simulink model "Power_split_controller"  (R2021b)
settings: Solver=VariableStepAuto  StartTime=0.0  StopTime=274  RelTol=1
undefined symbols (not defined in the file): ISOC_sy, Pd_SY, Pl_sy, Pu_sy, QC_sy, R0_sy, SOC_H, SOC_L, V0_sy
libraries: simulink x1
settings Model: Creator=bldha  LastModifiedBy=bldha
settings SolverCC: ZeroCrossAlgorithm=Adaptive
settings DebuggingCC: IgnoredZcDiagnostic=none

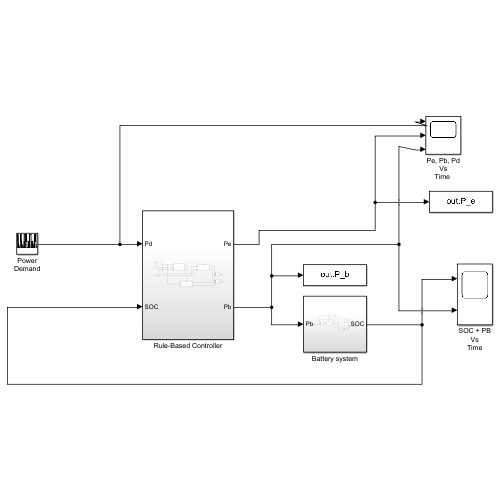
[thumbnail: Simulink's stored preview of the top-level diagram]
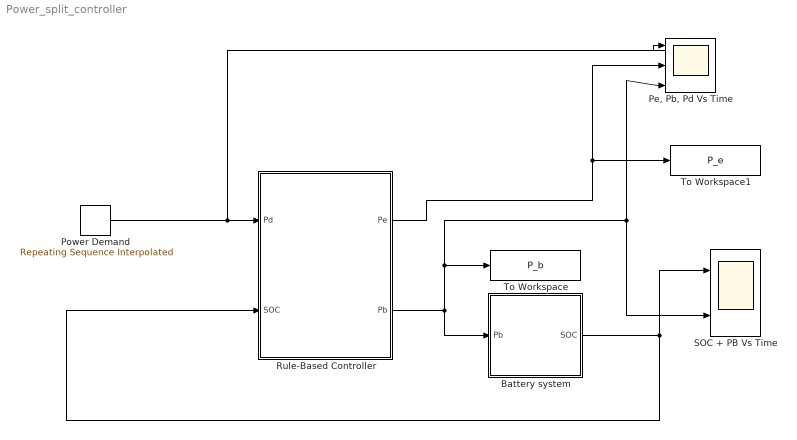
== system Power_split_controller ==
  Battery system : Subsystem
  "Pe, Pb, Pd Vs Time " : Scope  NumInputPorts=3
  Power Demand : simulink/Sources/Repeating Sequence Interpolated  OutValues=[Pd_SY.pow]  TimeValues=[Pd_SY.time]  LookUpMeth=Interpolation-Use End Values  tsamp=0.1  OutMin=[]  OutMax=[]  OutDataTypeStr=double  OutputDataTypeScalingMode=double  OutDataType=fixdt(0,8)  OutScaling=2^-10
  Rule-Based Controller : Subsystem
  SOC + PB Vs Time : Scope  NumInputPorts=2
  To Workspace : ToWorkspace  VariableName=P_b  SampleTime=-1
  To Workspace1 : ToWorkspace  VariableName=P_e  SampleTime=-1
  wires:
  Battery system/1(SOC) -> SOC + PB Vs Time/1, Rule-Based Controller/2(SOC)
  Rule-Based Controller/1(Pe) -> "Pe, Pb, Pd Vs Time "/2, To Workspace1/1
  Power Demand/1 -> Rule-Based Controller/1(Pd), "Pe, Pb, Pd Vs Time "/1
  Rule-Based Controller/2(Pb) -> To Workspace/1, "Pe, Pb, Pd Vs Time "/3, SOC + PB Vs Time/2, Battery system/1(Pb)

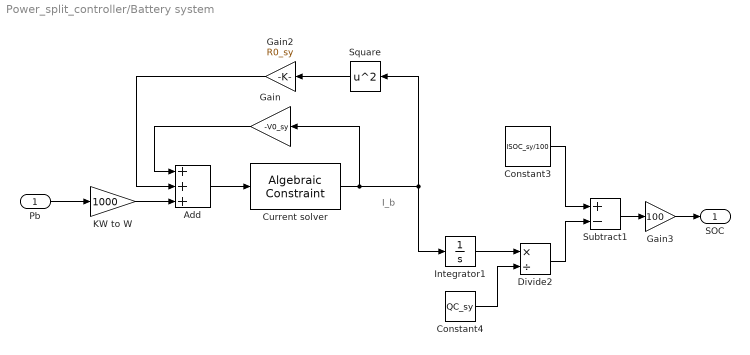
== system Power_split_controller/Battery system ==
  note: I_b
  Pb : Inport
  Add : Sum  Inputs=+++
  Constant3 : Constant  Value=ISOC_sy/100
  Constant4 : Constant  Value=QC_sy
  Current solver : AlgebraicConstraint  InitialGuess=-999999999999
  Divide2 : Product  Inputs=*/
  Gain : Gain  Gain=-V0_sy
  Gain2 : Gain  Gain=R0_sy
  Gain3 : Gain  Gain=100
  Integrator1 : Integrator
  KW to W : Gain  Gain=1000
  Square : Math  Operator=square  SaturateOnIntegerOverflow=on
  Subtract1 : Sum  Inputs=+-
  SOC : Outport
  wires:
  KW to W/1 -> Add/3
  Gain/1 -> Add/1
  Add/1 -> Current solver/1
  Square/1 -> Gain2/1
  Gain2/1 -> Add/2
  Pb/1 -> KW to W/1
  Divide2/1 -> Subtract1/2
  Constant3/1 -> Subtract1/1
  Subtract1/1 -> Gain3/1
  Gain3/1 -> SOC/1
  Current solver/1 -> Gain/1, Square/1, Integrator1/1
  Integrator1/1 -> Divide2/1
  Constant4/1 -> Divide2/2

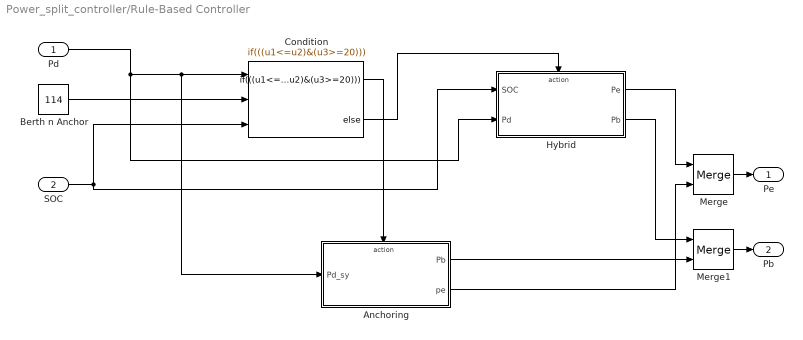
== system Power_split_controller/Rule-Based Controller ==
  Pd : Inport
  SOC : Inport  Port=2
  Anchoring : Subsystem  TreatAsAtomicUnit=on
  Berth n Anchor : Constant  Value=114
  Condition : If  NumInputs=3  IfExpression=((u1<=u2)&(u3>=20))
  Hybrid : Subsystem  TreatAsAtomicUnit=on
  Merge : Merge
  Merge1 : Merge
  Pe : Outport
  Pb : Outport  Port=2
  wires:
  Merge/1 -> Pe/1
  Pd/1 -> Hybrid/2(Pd), Anchoring/1(Pd_sy), Condition/1
  Berth n Anchor/1 -> Condition/2
  Anchoring/1(Pb) -> Merge1/2
  Hybrid/2(Pb) -> Merge1/1
  Merge1/1 -> Pb/1
  Hybrid/1(Pe) -> Merge/1
  Anchoring/2(pe) -> Merge/2
  SOC/1 -> Hybrid/1(SOC), Condition/3
  Condition/1 -> Anchoring/Action
  Condition/2 -> Hybrid/Action

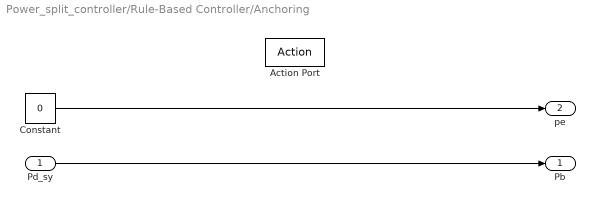
== system Power_split_controller/Rule-Based Controller/Anchoring ==
  Pd_sy : Inport
  Action Port : ActionPort  ActionPortLabel=if(((u1<=u2)&(u3>=20)))
  Constant : Constant  Value=0
  Pb : Outport
  pe : Outport  Port=2
  wires:
  Pd_sy/1 -> Pb/1
  Constant/1 -> pe/1

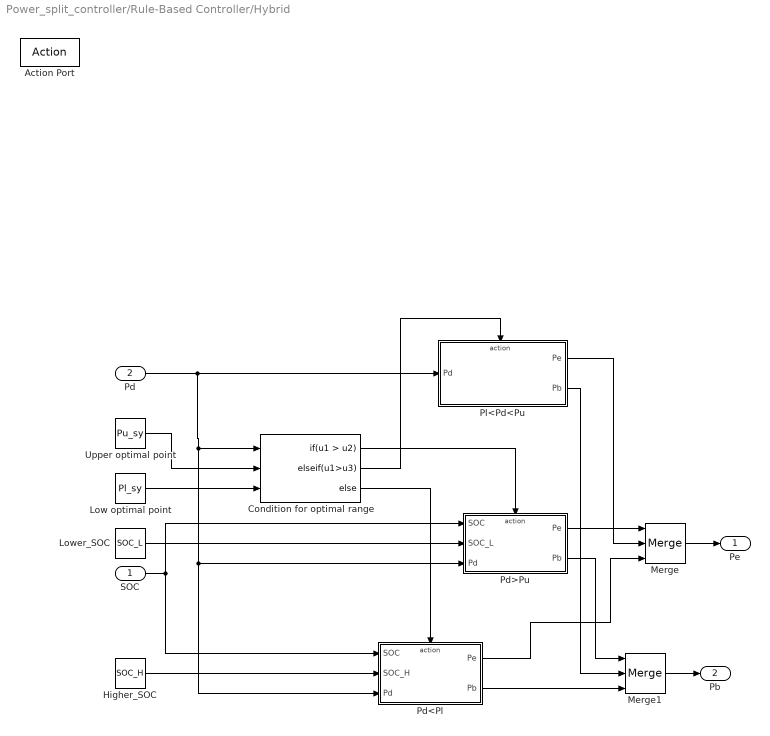
== system Power_split_controller/Rule-Based Controller/Hybrid ==
  SOC : Inport
  Pd : Inport  Port=2
  Action Port : ActionPort  ActionPortLabel=else
  "   Low optimal point" : Constant  Value=Pl_sy
  "  Upper optimal point " : Constant  Value=Pu_sy
  Condition for optimal range : If  NumInputs=3  IfExpression=u1 > u2  ElseIfExpressions=u1>u3
  Higher_SOC : Constant  Value=SOC_H
  Lower_SOC : Constant  Value=SOC_L
  Merge : Merge  Inputs=3
  Merge1 : Merge  Inputs=3
  Pd<Pl : Subsystem  TreatAsAtomicUnit=on
  Pd>Pu : Subsystem  TreatAsAtomicUnit=on
  Pl<Pd<Pu : Subsystem  TreatAsAtomicUnit=on
  Pe : Outport
  Pb : Outport  Port=2
  wires:
  Higher_SOC/1 -> Pd<Pl/2(SOC_H)
  Pl<Pd<Pu/2(Pb) -> Merge1/2
  Merge/1 -> Pe/1
  Pl<Pd<Pu/1(Pe) -> Merge/2
  Pd>Pu/2(Pb) -> Merge1/1
  Pd<Pl/1(Pe) -> Merge/3
  Lower_SOC/1 -> Pd>Pu/2(SOC_L)
  Pd/1 -> Pl<Pd<Pu/1(Pd), Pd<Pl/3(Pd), Pd>Pu/3(Pd), Condition for optimal range/1
  Condition for optimal range/2 -> Pl<Pd<Pu/Action
  Pd<Pl/2(Pb) -> Merge1/3
  "  Upper optimal point "/1 -> Condition for optimal range/2
  Condition for optimal range/3 -> Pd<Pl/Action
  Condition for optimal range/1 -> Pd>Pu/Action
  "   Low optimal point"/1 -> Condition for optimal range/3
  Pd>Pu/1(Pe) -> Merge/1
  Merge1/1 -> Pb/1
  SOC/1 -> Pd>Pu/1(SOC), Pd<Pl/1(SOC)

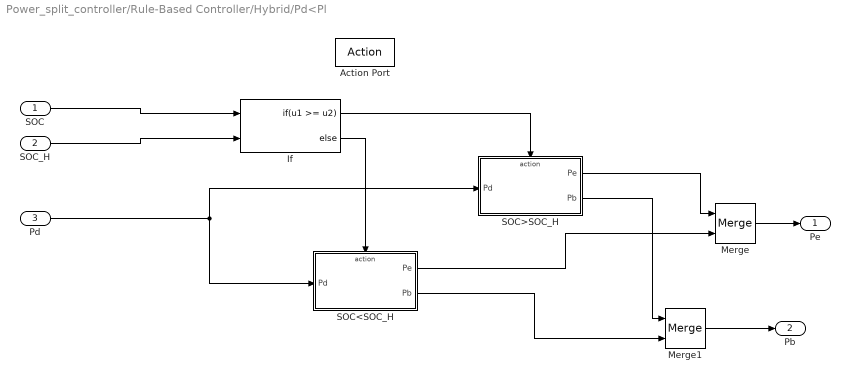
== system Power_split_controller/Rule-Based Controller/Hybrid/Pd<Pl ==
  SOC : Inport
  SOC_H : Inport  Port=2
  Pd : Inport  Port=3
  Action Port : ActionPort  ActionPortLabel=else
  If : If  NumInputs=2  IfExpression=u1 >= u2
  Merge : Merge
  Merge1 : Merge
  SOC<SOC_H : Subsystem  TreatAsAtomicUnit=on
  SOC>SOC_H : Subsystem  TreatAsAtomicUnit=on
  Pe : Outport
  Pb : Outport  Port=2
  wires:
  SOC/1 -> If/1
  SOC_H/1 -> If/2
  SOC>SOC_H/1(Pe) -> Merge/1
  SOC<SOC_H/1(Pe) -> Merge/2
  Merge/1 -> Pe/1
  SOC>SOC_H/2(Pb) -> Merge1/1
  SOC<SOC_H/2(Pb) -> Merge1/2
  Merge1/1 -> Pb/1
  Pd/1 -> SOC<SOC_H/1(Pd), SOC>SOC_H/1(Pd)
  If/2 -> SOC<SOC_H/Action
  If/1 -> SOC>SOC_H/Action

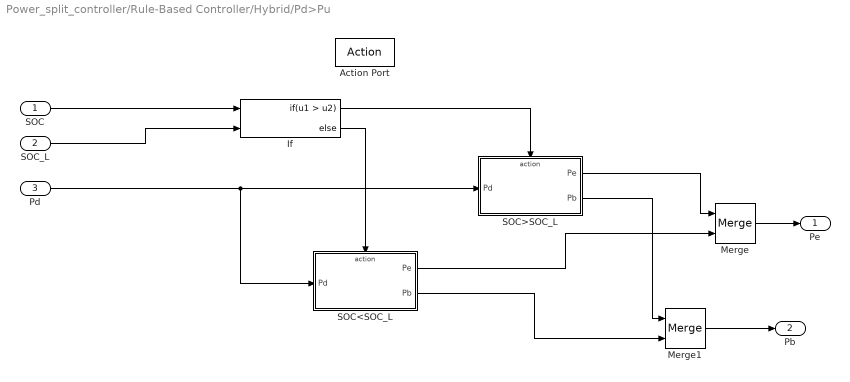
== system Power_split_controller/Rule-Based Controller/Hybrid/Pd>Pu ==
  SOC : Inport
  SOC_L : Inport  Port=2
  Pd : Inport  Port=3
  Action Port : ActionPort  ActionPortLabel=if(u1 > u2)
  If : If  NumInputs=2  IfExpression=u1 > u2
  Merge : Merge
  Merge1 : Merge
  SOC<SOC_L : Subsystem  TreatAsAtomicUnit=on
  SOC>SOC_L : Subsystem  TreatAsAtomicUnit=on
  Pe : Outport
  Pb : Outport  Port=2
  wires:
  SOC/1 -> If/1
  SOC_L/1 -> If/2
  If/1 -> SOC>SOC_L/Action
  If/2 -> SOC<SOC_L/Action
  SOC>SOC_L/1(Pe) -> Merge/1
  SOC<SOC_L/1(Pe) -> Merge/2
  Merge/1 -> Pe/1
  SOC>SOC_L/2(Pb) -> Merge1/1
  SOC<SOC_L/2(Pb) -> Merge1/2
  Merge1/1 -> Pb/1
  Pd/1 -> SOC<SOC_L/1(Pd), SOC>SOC_L/1(Pd)

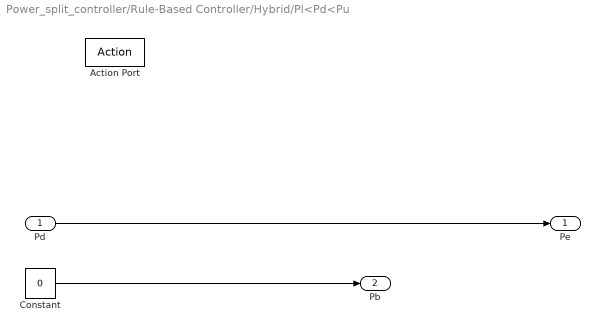
== system Power_split_controller/Rule-Based Controller/Hybrid/Pl<Pd<Pu ==
  Pd : Inport
  Action Port : ActionPort  ActionPortLabel=elseif(u1>u3)
  Constant : Constant  Value=0
  Pe : Outport
  Pb : Outport  Port=2
  wires:
  Pd/1 -> Pe/1
  Constant/1 -> Pb/1

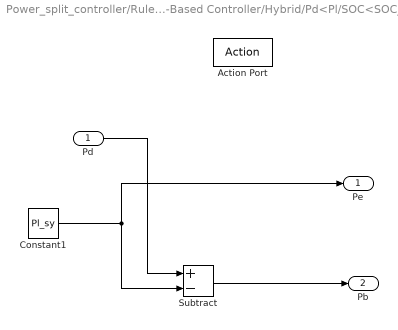
== system Power_split_controller/Rule-Based Controller/Hybrid/Pd<Pl/SOC<SOC_H ==
  Pd : Inport
  Action Port : ActionPort  ActionPortLabel=else
  Constant1 : Constant  Value=Pl_sy
  Subtract : Sum  Inputs=+-
  Pe : Outport
  Pb : Outport  Port=2
  wires:
  Pd/1 -> Subtract/1
  Constant1/1 -> Pe/1, Subtract/2
  Subtract/1 -> Pb/1

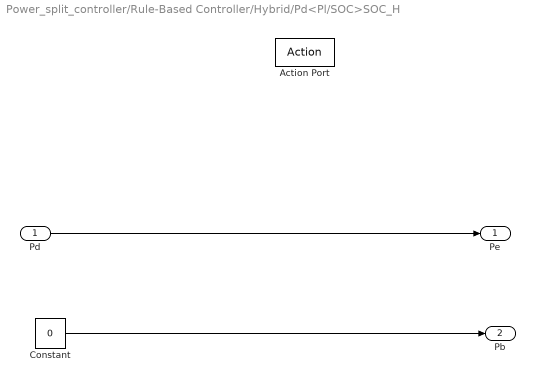
== system Power_split_controller/Rule-Based Controller/Hybrid/Pd<Pl/SOC>SOC_H ==
  Pd : Inport
  Action Port : ActionPort  ActionPortLabel=if(u1 >= u2)
  Constant : Constant  Value=0
  Pe : Outport
  Pb : Outport  Port=2
  wires:
  Pd/1 -> Pe/1
  Constant/1 -> Pb/1

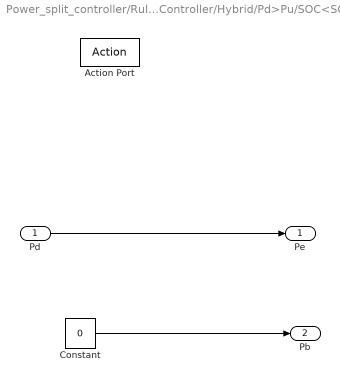
== system Power_split_controller/Rule-Based Controller/Hybrid/Pd>Pu/SOC<SOC_L ==
  Pd : Inport
  Action Port : ActionPort  ActionPortLabel=else
  Constant : Constant  Value=0
  Pe : Outport
  Pb : Outport  Port=2
  wires:
  Constant/1 -> Pb/1
  Pd/1 -> Pe/1

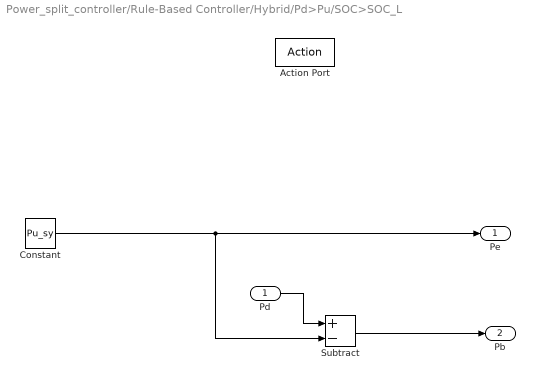
== system Power_split_controller/Rule-Based Controller/Hybrid/Pd>Pu/SOC>SOC_L ==
  Pd : Inport
  Action Port : ActionPort  ActionPortLabel=if(u1 > u2)
  Constant : Constant  Value=Pu_sy
  Subtract : Sum  Inputs=+-
  Pe : Outport
  Pb : Outport  Port=2
  wires:
  Constant/1 -> Subtract/2, Pe/1
  Pd/1 -> Subtract/1
  Subtract/1 -> Pb/1
